simulink model "verified_components"  (R2021b)
settings: Solver=VariableStepAuto  StartTime=0.0  StopTime=250  RelTol=1e-3
undefined symbols (not defined in the file or in its folder): F, HDBK, Light, MIL, STD
libraries: aerolibatmos2 x4, aerolibwind2 x2, simulink x2, shared6dof x1
settings Model: Creator=zhongyuliang  LastModifiedBy=zhongyuliang

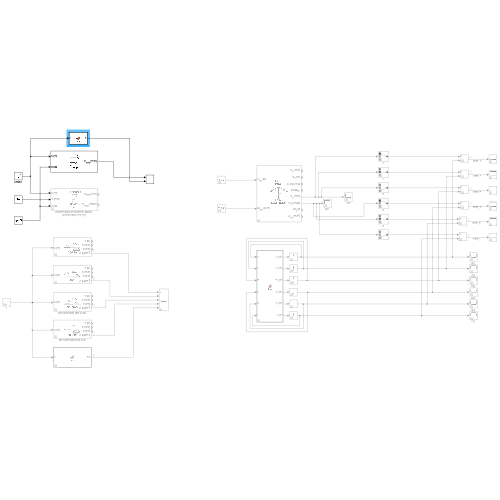
[thumbnail: Simulink's stored preview of the top-level diagram]
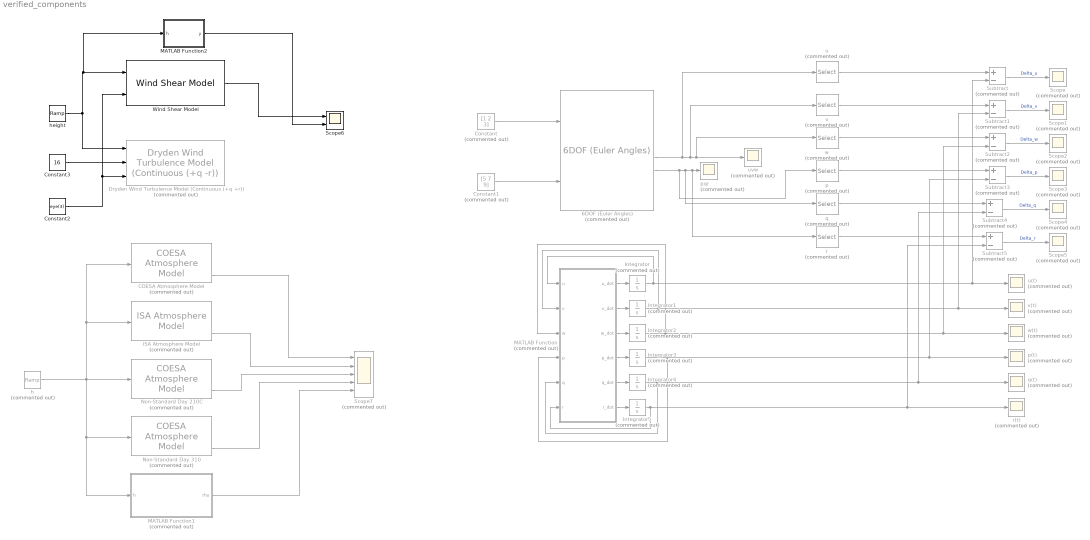
== system verified_components ==
  6DOF (Euler Angles) : shared6dof/6DOF (Euler Angles)  Commented=on  units=Metric (MKS)  mtype=Fixed  rep=Euler Angles  xme_0=[0 0 0]  Vm_0=[0 0 0]  eul_0=[0 0 0]  pm_0=[0 0 0]  mass_0=1  mass_e=0.5  mass_f=2.0  inertia=|  inertia_e=eye(3)  inertia_f=2*eye(3)  k_quat=1.0  vre_flag=on  abi_flag=off  aMode=0  xme_statename=''  Vm_statename=''  eul_statename=''  quat_statename=''  pm_statename=''  mass_statename=''
      | [3.14, 2.17, 1.58;
      |          2.17, 5.12 ,6.44;
      |          1.58 ,6.44 ,9.75]
      settings: SourceProductBaseCode=AE,PW,DR,MT,UV,VE
  COESA Atmosphere Model : aerolibatmos2/COESA Atmosphere Model  Commented=on  units=Metric (MKS)  spec=1976 COESA-extended U.S. Standard Atmosphere  model=Profile  profile_var=High temperature  profile_percent=1%  profile_alt=5 km (16404 ft)  envelope_var=High temperature  envelope_percent=1%  action=Warning
  Constant : Constant  Commented=on  Value=[1 2 3]
  Constant1 : Constant  Commented=on  Value=[5 7 9]
  Constant2 : Constant  Value=eye(3)
  Constant3 : Constant  Value=16
  Dryden Wind Turbulence Model (Continuous (+q +r)) : aerolibwind2/Dryden Wind Turbulence Model  (Continuous (+q -r))  Commented=on  units=Metric (MKS)  spec=MIL-F-8785C  model=Continuous Dryden (+q +r)  W20=turbulence_vel_at6m  Wdeg=turbulence_ori_at6m  TurbProb=10^-2 - Light  L_high=533.4  Wingspan=10  ts=0.1  Seed=[23341 23342 23343 23344]  T_on=on
  ISA Atmosphere Model : aerolibatmos2/ISA Atmosphere Model  Commented=on  custom=off  g=9.80665  gamma=1.4  R=287.0531  L=0.0065  h_trop=11000  h_strat=20000  rho0=1.225  P0=101325  T0=288.15  h0=0
  Integrator{,1..5} (6 alike) : Integrator  Commented=on
  MATLAB Function : MATLAB Function  Commented=on  TreatAsAtomicUnit=on
  MATLAB Function1 : MATLAB Function  Commented=on  TreatAsAtomicUnit=on
  MATLAB Function2 : MATLAB Function  TreatAsAtomicUnit=on
  Non-Standard Day 210C : aerolibatmos2/COESA Atmosphere Model  Commented=on  units=Metric (MKS)  spec=MIL-STD-210C  model=Profile  profile_var=High temperature  profile_percent=1%  profile_alt=5 km (16404 ft)  envelope_var=High temperature  envelope_percent=1%  action=Warning
  Non-Standard Day 310 : aerolibatmos2/COESA Atmosphere Model  Commented=on  units=Metric (MKS)  spec=MIL-HDBK-310  model=Profile  profile_var=High temperature  profile_percent=1%  profile_alt=5 km (16404 ft)  envelope_var=High temperature  envelope_percent=1%  action=Warning
  Scope{,1..5} (6 alike) : Scope  Commented=on
  Scope6 : Scope  NumInputPorts=2
  Scope7 : Scope  Commented=on  NumInputPorts=5
  Subtract{,1..5} (6 alike) : Sum  Commented=on  Inputs=+-
  Wind Shear Model : aerolibwind2/Wind Shear Model  units=Metric (MKS)  phase=Category C - Terminal Flight Phase  W_20=1.5  Wdeg=180
  h : simulink/Sources/Ramp  Commented=on  slope=1  start=0  InitialOutput=0
  height : simulink/Sources/Ramp  slope=1  start=0  InitialOutput=0
  p : Selector  Commented=on  InputPortWidth=3  IndexOptions=Index vector (dialog)  Indices=1  OutputSizes=1
  p(t) : Scope  Commented=on
  pqr : Scope  Commented=on
  q : Selector  Commented=on  InputPortWidth=3  IndexOptions=Index vector (dialog)  Indices=2  OutputSizes=1
  q(t) : Scope  Commented=on
  r : Selector  Commented=on  InputPortWidth=3  IndexOptions=Index vector (dialog)  Indices=3  OutputSizes=1
  r(t) : Scope  Commented=on
  u : Selector  Commented=on  InputPortWidth=3  IndexOptions=Index vector (dialog)  Indices=1  OutputSizes=1
  u(t) : Scope  Commented=on
  uvw : Scope  Commented=on
  v : Selector  Commented=on  InputPortWidth=3  IndexOptions=Index vector (dialog)  Indices=2  OutputSizes=1
  v(t) : Scope  Commented=on
  w : Selector  Commented=on  InputPortWidth=3  IndexOptions=Index vector (dialog)  Indices=3  OutputSizes=1
  w(t) : Scope  Commented=on
  wires:
  MATLAB Function/1(u_dot) -> Integrator/1
  MATLAB Function/2(v_dot) -> Integrator1/1
  MATLAB Function/4(p_dot) -> Integrator3/1
  MATLAB Function/6(r_dot) -> Integrator5/1
  MATLAB Function/5(q_dot) -> Integrator4/1
  MATLAB Function/3(w_dot) -> Integrator2/1
  Integrator1/1 -> Subtract1/2, v(t)/1, MATLAB Function/2(v)
  Integrator2/1 -> MATLAB Function/3(w), Subtract2/2, w(t)/1
  Integrator5/1 -> MATLAB Function/6(r), Subtract5/2, r(t)/1
  Integrator4/1 -> MATLAB Function/5(q), Subtract4/2, q(t)/1
  Constant/1 -> 6DOF (Euler Angles)/1
  6DOF (Euler Angles)/5 -> u/1, v/1, uvw/1, w/1
  6DOF (Euler Angles)/6 -> p/1, q/1, r/1, pqr/1
  Integrator/1 -> MATLAB Function/1(u), Subtract/2, u(t)/1
  Integrator3/1 -> MATLAB Function/4(p), Subtract3/2, p(t)/1
  Constant1/1 -> 6DOF (Euler Angles)/2
  u/1 -> Subtract/1
  r/1 -> Subtract5/1
  q/1 -> Subtract4/1
  p/1 -> Subtract3/1
  w/1 -> Subtract2/1
  v/1 -> Subtract1/1
  Subtract/1 -> Scope/1  "Delta_u"
  Subtract1/1 -> Scope1/1  "Delta_v"
  Subtract2/1 -> Scope2/1  "Delta_w"
  Subtract3/1 -> Scope3/1  "Delta_p"
  Subtract4/1 -> Scope4/1  "Delta_q"
  Subtract5/1 -> Scope5/1  "Delta_r"
  height/1 -> Dryden Wind Turbulence Model (Continuous (+q +r))/1, MATLAB Function2/1(h), Wind Shear Model/1
  Wind Shear Model/1 -> Scope6/1
  Constant3/1 -> Dryden Wind Turbulence Model (Continuous (+q +r))/2
  Constant2/1 -> Wind Shear Model/2, Dryden Wind Turbulence Model (Continuous (+q +r))/3
  Non-Standard Day 210C/4 -> Scope7/3
  Non-Standard Day 310/4 -> Scope7/4
  ISA Atmosphere Model/4 -> Scope7/2
  MATLAB Function1/1(rho) -> Scope7/5
  COESA Atmosphere Model/4 -> Scope7/1
  h/1 -> ISA Atmosphere Model/1, COESA Atmosphere Model/1, MATLAB Function1/1(h), Non-Standard Day 310/1, Non-Standard Day 210C/1
  MATLAB Function2/1(y) -> Scope6/2

== matlab function verified_components/MATLAB Function1 ==
  data: h input; rho output
function rho = fcn(h)
    c_h = 1.225;
    c_z = 2.256e-5;
    c_e = 4.2559;
    rho = c_h*(1 - h*c_z)^(c_e);
end

== matlab function verified_components/MATLAB Function ==
  data: u input; u_dot output; v input; w input; p input; q input; r input; v_dot output; w_dot output; p_dot output; q_dot output; r_dot output
function [u_dot, v_dot, w_dot, p_dot, q_dot, r_dot] = fcn(u,v,w,p,q,r)
    B_F = [1;2;3];
    m = 1;
    B_M = [5;7;9];
    I = [3.14, 2.17, 1.58;
         2.17, 5.12, 6.44;
         1.58, 6.44, 9.75];

    uvw = -skew([p;q;r;])*[u;v;w;] + B_F/m;
    u_dot = uvw(1);
    v_dot = uvw(2);
    w_dot = uvw(3);

    pqr = I\(B_M - skew([p;q;r])*I*[p;q;r]);
    p_dot = pqr(1);
    q_dot = pqr(2);
    r_dot = pqr(3);
end

function M = skew(a)
    M = [0,     -a(3), a(2);
         a(3),  0    , -a(1);
         -a(2), a(1) , 0];
end

== matlab function verified_components/MATLAB Function2 ==
  data: h input; y output
function y = fcn(h)

y = (h>0.04572)*1.5*log(h/0.04572)/log(6.096/0.04572);
